simulink model "sedemo_rtos_application"  (Simulink 7.5)
settings: Solver=VariableStepDiscrete  StartTime=0.0  StopTime=19  MaxStep=inf  RelTol=1e-3
undefined symbols (not defined in the file or in its folder): des_figposition
libraries: simeventssink1 x12, simeventsgenerators1 x9, simeventsrouting1 x6, simulink x6, simeventsattributes2 x5, simeventstranslate1 x4, simeventsinfo x1, simeventsserver1 x1, simeventsqueue1 x1
settings Model: Creator=The MathWorks Inc.  ExtModeAutoUpdateStatusClock=off
settings SolverCC: InsertRTBMode=Auto
settings OptimizationCC: InitFltsAndDblsToZero=on
settings DebuggingCC: ReadBeforeWriteMsg=DisableAll  WriteAfterWriteMsg=DisableAll  WriteAfterReadMsg=DisableAll  SaveWithParameterizedLinksMsg=none  SignalResolutionControl=TryResolveAllWithWarning  MultiTaskDSMMsg=warning  MultiTaskCondExecSysMsg=none  StrictBusMsg=Warning
settings RTWCC: IncludeERTFirstTime=on
settings GRTTargetCC: TargetFcnLib=ansi_tfl_tmw.mat
settings SimEventsCC: propDiagAttribOutput=1  propDiagFcnCallOutput=1  propDiagStatOutput=0

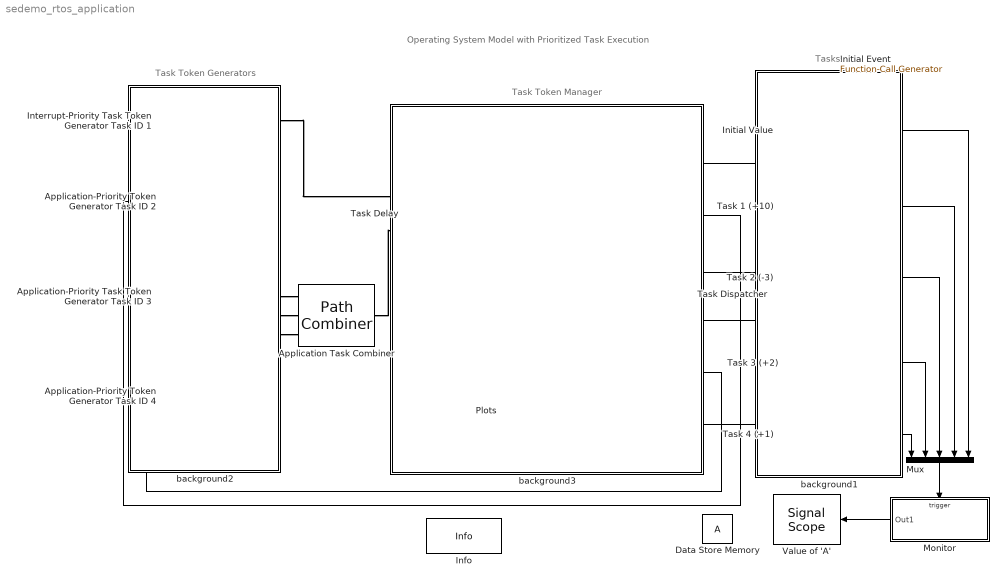
== system sedemo_rtos_application ==
  note: Operating System Model with Prioritized Task Execution
  note: Task Token Generators
  note: Task Token Manager
  note: Tasks
  Application Task Combiner : simeventsrouting1/Path Combiner  Priority=1  SystemSampleTime=-1  NumberInputPorts=3  InputPortPrecedence=IN1 port  InitialSeed=45675  SpecifyEventPriority=off  PriorityPathCombinerPortPrecedenceSelection=4100  StatNumberDeparted=Off  StatLastArrivalPort=Off  EvaluatedNumPorts=3
  Application-Priority Token Generator Task ID 2 : Subsystem
  Application-Priority Token Generator Task ID 4 : Subsystem
  Application-Priority Task Token Generator Task ID 3 : Subsystem
  Data Store Memory : DataStoreMemory  DataStoreName=A  ReadBeforeWriteMsg=warning  WriteAfterWriteMsg=warning  WriteAfterReadMsg=warning  OutDataType=sfix(16)  OutScaling=2^0
  Info : simeventsinfo/Info  SystemSampleTime=-1
  Initial Event : simulink/Ports & Subsystems/Function-Call Generator  sample_time=1e20  numberOfIterations=1
  Initial Value : Subsystem  TreatAsAtomicUnit=on
  Interrupt-Priority Task Token Generator Task ID 1 : Subsystem
  Monitor : Subsystem  TreatAsAtomicUnit=on
      settings: PropExecContextOutsideSubsystem=on
  Mux : Mux  Inputs=5
  Plots : Subsystem
  Task 1 (+10) : Subsystem  TreatAsAtomicUnit=on
  Task 2 (-3) : Subsystem  TreatAsAtomicUnit=on
  Task 3 (+2) : Subsystem  TreatAsAtomicUnit=on
  Task 4 (+1) : Subsystem  TreatAsAtomicUnit=on
  Task Delay : Subsystem
  Task Dispatcher : Subsystem
  Value of 'A' : simeventssink1/Signal Scope  Priority=1  SystemSampleTime=-1  PlotType=Stair  InputType=Signal  NumInputs=1  AttributeNameY=Count  XInputOptionSignal=Event time  XInputOptionEntity=Event time  AttributeNameX=Count  EnableEntityOutport=on  XMin=0  XMax=15.5  XLimitExceededOption=Stretch axis limits  YLimitExceededOption=Stretch axis limits  AxisGrid=on  AxisLegend=off  LineDisables=""  LineColors=b  LineStyles=-  LineMarkers=.  OpenScopeAtSimStart=on  Title=Value of 'A'  YLabel='A'  XLabel=Time  FigurePosition=des_figposition([74 15 24 20])  AxisZoom=off  DataStoreOption=Limited  DataPointsLimit=10000  StatNumberArrived=Off  ShowCountPlotted=off  ShowToolbar=off
      settings: YMin=-0.25  YMax=27
  background1 : Subsystem
      mask Display: disp('')
  background2 : Subsystem
      mask Display: disp('')
  background3 : Subsystem
      mask Display: disp('')
  wires:
  Task Dispatcher/3(Task 2) -> Task 2 (-3)/Trigger
  Task Dispatcher/4(Task 3) -> Task 3 (+2)/Trigger
  Mux/1 -> Monitor/Trigger
  Task 3 (+2)/1(Out1) -> Mux/2
  Task 2 (-3)/1(Out1) -> Mux/3
  Task 1 (+10)/1(Out1) -> Mux/4
  Task 4 (+1)/1(Out1) -> Mux/1
  Initial Value/1(Out1) -> Mux/5
  Task Dispatcher/2(Next task 1) -> Application-Priority Token Generator Task ID 2/1(Start)
  Initial Event/1 -> Initial Value/Trigger
  Task Dispatcher/1(Task 1) -> Task 1 (+10)/Trigger
  Task Dispatcher/6(Task 4) -> Task 4 (+1)/Trigger
  Task Dispatcher/5(Next task 3) -> Application-Priority Token Generator Task ID 4/1(Start)
  Monitor/1(Out1) -> Value of 'A'/1
  connections:
  Interrupt-Priority Task Token Generator Task ID 1/RConn1 -- Task Delay/LConn1
  Application-Priority Token Generator Task ID 2/RConn1 -- Application Task Combiner/LConn3
  Task Dispatcher/LConn2 -- Plots/LConn1
  Task Delay/RConn1 -- Task Dispatcher/LConn1
  Application-Priority Task Token Generator Task ID 3/RConn1 -- Application Task Combiner/LConn1
  Application-Priority Token Generator Task ID 4/RConn1 -- Application Task Combiner/LConn2
  Application Task Combiner/RConn1 -- Task Delay/LConn2

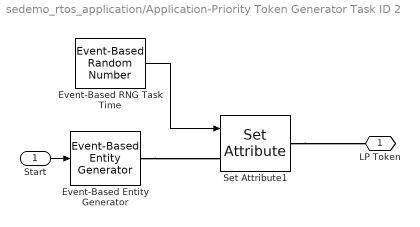
== system sedemo_rtos_application/Application-Priority Token Generator Task ID 2 ==
  Start : Inport  OutDataType=sfix(16)  OutScaling=2^0
  Event-Based Entity Generator : simeventsgenerators1/Entity Generators/Event-Based Entity Generator  Priority=1  DialogController=des_ddg_create  DialogControllerArgs=DataTag2  SystemSampleTime=-1  GenerateEntitiesUpon=Function call from port fcn  SignalEdgeType=Rising  SpecifyEventPriority=on  PriorityEntityGeneration=301  GenerateEntityAtSimulationStart=on  AllowBlocking=on  ResponseDuringBlockage=Discard generated entities  EntityType=Standard  StatNumberDeparted=Off  StatPendingEntity=Off  StatAverageIntergenerationTime=Off
  Event-Based RNG Task Time : simeventsgenerators1/Signal Generators/Event-Based Random Number  SystemSampleTime=-1  distribution=Uniform  meanExp=2  minUnif=1  maxUnif=1  pOneBern=0.25  pSuccessBino=0.5  numTrialBino=1  meanNorm=0  stdNorm=1  minTri=1  maxTri=3  modeTri=2  thresholdLogn=0  scaleLogn=1  shapeLogn=1  pSuccessGeo=0.5  meanPoiss=1  thresholdLogl=0  scaleLogl=1  thresholdGam=0  scaleGam=1  shapeGam=1  minBeta=0  maxBeta=1  shape1Beta=1  shape2Beta=1  minUnid=0  maxUnid=1  numValueUnid=2  thresholdWbl=0  scaleWbl=1  shapeWbl=1  valueVecCont=[0 1]  cdfVecCont=[0 1]  valueVecDisc=[0 1]  probVecDisc=[0.5 0.5]  seed=2354676  IsProcessed=on  isConnected=1
  Set Attribute1 : simeventsattributes2/Set Attribute  Priority=1  DialogController=des_ddg_create  DialogControllerArgs=DataTag4  SystemSampleTime=-1  AttributeFrom=Dialog|Signal port|Dialog|Dialog  AttributeName=PriorityAttributeName|TaskExecTime|TaskType|TaskID  AttributeTreatAsVector=1|1|1|1  AttributeValue=2|1|2|2  AttributeCreate=on  StatNumberDeparted=Off  EvaluatedAttributeValue={2;[];2;2}
  LP Token : PMIOPort  Port=1  Side=Right
  wires:
  Event-Based RNG Task Time/1 -> Set Attribute1/1
  Start/1 -> Event-Based Entity Generator/1
  connections:
  Event-Based Entity Generator/RConn1 -- Set Attribute1/LConn1
  Set Attribute1/RConn1 -- LP Token/RConn1

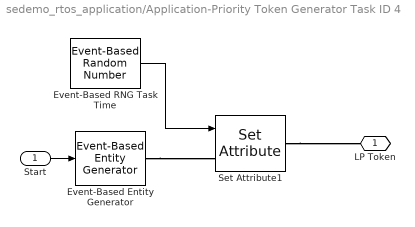
== system sedemo_rtos_application/Application-Priority Token Generator Task ID 4 ==
  Start : Inport  OutDataType=sfix(16)  OutScaling=2^0
  Event-Based Entity Generator : simeventsgenerators1/Entity Generators/Event-Based Entity Generator  Priority=1  DialogController=des_ddg_create  DialogControllerArgs=DataTag6  SystemSampleTime=-1  GenerateEntitiesUpon=Function call from port fcn  SignalEdgeType=Rising  SpecifyEventPriority=on  PriorityEntityGeneration=299  GenerateEntityAtSimulationStart=on  AllowBlocking=on  ResponseDuringBlockage=Discard generated entities  EntityType=Standard  StatNumberDeparted=Off  StatPendingEntity=Off  StatAverageIntergenerationTime=Off
  Event-Based RNG Task Time : simeventsgenerators1/Signal Generators/Event-Based Random Number  SystemSampleTime=-1  distribution=Uniform  meanExp=2  minUnif=2  maxUnif=2  pOneBern=0.25  pSuccessBino=0.5  numTrialBino=1  meanNorm=0  stdNorm=1  minTri=1  maxTri=3  modeTri=2  thresholdLogn=0  scaleLogn=1  shapeLogn=1  pSuccessGeo=0.5  meanPoiss=1  thresholdLogl=0  scaleLogl=1  thresholdGam=0  scaleGam=1  shapeGam=1  minBeta=0  maxBeta=1  shape1Beta=1  shape2Beta=1  minUnid=0  maxUnid=1  numValueUnid=2  thresholdWbl=0  scaleWbl=1  shapeWbl=1  valueVecCont=[0 1]  cdfVecCont=[0 1]  valueVecDisc=[0 1]  probVecDisc=[0.5 0.5]  seed=675409  IsProcessed=on  isConnected=1
  Set Attribute1 : simeventsattributes2/Set Attribute  Priority=1  DialogController=des_ddg_create  DialogControllerArgs=DataTag8  SystemSampleTime=-1  AttributeFrom=Dialog|Signal port|Dialog|Dialog  AttributeName=PriorityAttributeName|TaskExecTime|TaskType|TaskID  AttributeTreatAsVector=1|1|1|1  AttributeValue=4|1|2|4  AttributeCreate=on  StatNumberDeparted=Off  EvaluatedAttributeValue={4;[];2;4}
  LP Token : PMIOPort  Port=1  Side=Right
  wires:
  Event-Based RNG Task Time/1 -> Set Attribute1/1
  Start/1 -> Event-Based Entity Generator/1
  connections:
  Event-Based Entity Generator/RConn1 -- Set Attribute1/LConn1
  Set Attribute1/RConn1 -- LP Token/RConn1

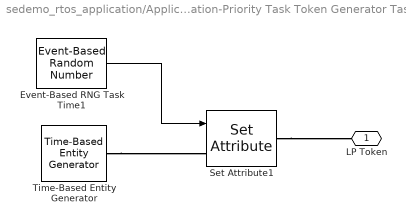
== system sedemo_rtos_application/Application-Priority Task Token Generator Task ID 3 ==
  Event-Based RNG Task Time1 : simeventsgenerators1/Signal Generators/Event-Based Random Number  SystemSampleTime=-1  distribution=Uniform  meanExp=2  minUnif=1.5  maxUnif=1.5  pOneBern=0.25  pSuccessBino=0.5  numTrialBino=1  meanNorm=0  stdNorm=1  minTri=1  maxTri=3  modeTri=2  thresholdLogn=0  scaleLogn=1  shapeLogn=1  pSuccessGeo=0.5  meanPoiss=1  thresholdLogl=0  scaleLogl=1  thresholdGam=0  scaleGam=1  shapeGam=1  minBeta=0  maxBeta=1  shape1Beta=1  shape2Beta=1  minUnid=0  maxUnid=1  numValueUnid=2  thresholdWbl=0  scaleWbl=1  shapeWbl=1  valueVecCont=[0 1]  cdfVecCont=[0 1]  valueVecDisc=[0 1]  probVecDisc=[0.5 0.5]  seed=6532180  IsProcessed=on  isConnected=1
  Set Attribute1 : simeventsattributes2/Set Attribute  Priority=1  DialogController=des_ddg_create  DialogControllerArgs=DataTag10  SystemSampleTime=-1  AttributeFrom=Dialog|Signal port|Dialog|Dialog  AttributeName=PriorityAttributeName|TaskExecTime|TaskType|TaskID  AttributeTreatAsVector=1|1|1|1  AttributeValue=3|1|2|3  AttributeCreate=on  StatNumberDeparted=Off  EvaluatedAttributeValue={3;[];2;3}
  Time-Based Entity Generator : simeventsgenerators1/Entity Generators/Time-Based Entity Generator  Priority=1  DialogController=des_ddg_create  DialogControllerArgs=DataTag12  SystemSampleTime=-1  GenerateEntitiesUpon=Intergeneration time from dialog  Distribution=Constant  Minimum=9.9  Maximum=10.5  Mean=10  InitialSeed=12345  Period=9.9  PriorityEntityGeneration=290  GenerateEntityAtSimulationStart=on  ResponseWhenBlocked=Pause generation  ResponseWhenUnblocked=Immediate restart  EntityType=Standard  StatNumberDeparted=Off  StatPendingEntity=Off  StatAverageIntergenerationTime=Off
  LP Token : PMIOPort  Port=1  Side=Right
  wires:
  Event-Based RNG Task Time1/1 -> Set Attribute1/1
  connections:
  Time-Based Entity Generator/RConn1 -- Set Attribute1/LConn1
  Set Attribute1/RConn1 -- LP Token/RConn1

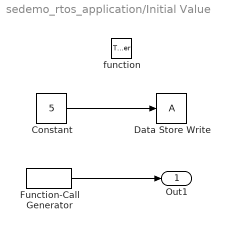
== system sedemo_rtos_application/Initial Value ==
  function : TriggerPort  TriggerType=function-call
  Constant : Constant  Value=5  OutDataType=sfix(16)  OutScaling=2^0
  Data Store Write : DataStoreWrite  DataStoreName=A  SampleTime=-1
  Function-Call Generator : simulink/Ports & Subsystems/Function-Call Generator  sample_time=-1  numberOfIterations=1
  Out1 : Outport  OutDataType=sfix(16)  OutScaling=2^0
  wires:
  Constant/1 -> Data Store Write/1
  Function-Call Generator/1 -> Out1/1

== system sedemo_rtos_application/Interrupt-Priority Task Token Generator Task ID 1 ==
  Event-Based RNG Task Time : simeventsgenerators1/Signal Generators/Event-Based Random Number  SystemSampleTime=-1  distribution=Uniform  meanExp=0.9  minUnif=.45  maxUnif=.45  pOneBern=0.25  pSuccessBino=0.5  numTrialBino=1  meanNorm=0  stdNorm=1  minTri=1  maxTri=3  modeTri=2  thresholdLogn=0  scaleLogn=1  shapeLogn=1  pSuccessGeo=0.5  meanPoiss=1  thresholdLogl=0  scaleLogl=1  thresholdGam=0  scaleGam=1  shapeGam=1  minBeta=0  maxBeta=1  shape1Beta=1  shape2Beta=1  minUnid=0  maxUnid=1  numValueUnid=2  thresholdWbl=0  scaleWbl=1  shapeWbl=1  valueVecCont=[0 1]  cdfVecCont=[0 1]  valueVecDisc=[0 1]  probVecDisc=[0.5 0.5]  seed=25899  IsProcessed=on  isConnected=1
  Set Attribute : simeventsattributes2/Set Attribute  Priority=1  DialogController=des_ddg_create  DialogControllerArgs=DataTag14  SystemSampleTime=-1  AttributeFrom=Dialog|Signal port|Dialog|Dialog  AttributeName=PriorityAttributeName|TaskExecTime|TaskType|TaskID  AttributeTreatAsVector=1|1|1|1  AttributeValue=1|1|2|1  AttributeCreate=on  StatNumberDeparted=Off  EvaluatedAttributeValue={1;[];2;1}
  Time-Based Entity Generator : simeventsgenerators1/Entity Generators/Time-Based Entity Generator  Priority=1  DialogController=des_ddg_create  DialogControllerArgs=DataTag16  SystemSampleTime=-1  GenerateEntitiesUpon=Intergeneration time from dialog  Distribution=Constant  Minimum=0  Maximum=1  Mean=1  InitialSeed=12345  Period=10  PriorityEntityGeneration=1  GenerateEntityAtSimulationStart=on  ResponseWhenBlocked=Pause generation  ResponseWhenUnblocked=Immediate restart  EntityType=Standard  StatNumberDeparted=Off  StatPendingEntity=Off  StatAverageIntergenerationTime=Off
  HP Token : PMIOPort  Port=1  Side=Right
  wires:
  Event-Based RNG Task Time/1 -> Set Attribute/1
  connections:
  Set Attribute/RConn1 -- HP Token/RConn1
  Time-Based Entity Generator/RConn1 -- Set Attribute/LConn1

== system sedemo_rtos_application/Monitor ==
  function : TriggerPort  TriggerType=function-call
  Data Store Read : DataStoreRead  DataStoreName=A  SampleTime=-1
  Out1 : Outport  OutDataType=sfix(16)  OutScaling=2^0
  wires:
  Data Store Read/1 -> Out1/1

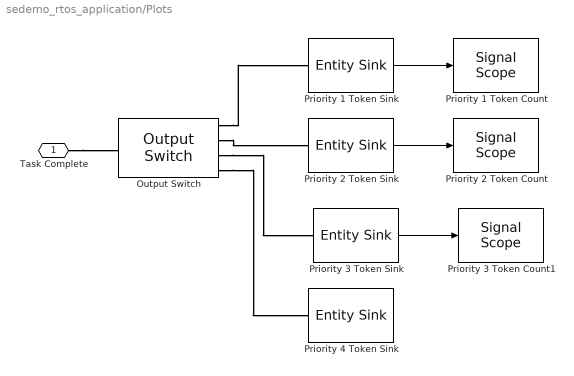
== system sedemo_rtos_application/Plots ==
  Output Switch : simeventsrouting1/Output Switch  Priority=1  SystemSampleTime=-1  NumberOutputPorts=4  SwitchingCriterion=From attribute  InitialSeed=34567  AttributeName=PriorityAttributeName  InitialConditionsOpt=off  InitialConditions=1  EntityBufferOpt=off  SpecifyEventPriority=off  PriorityOutputSwitchSelectPort=4100  TimeoutPortOpt=off  StatNumberDeparted=Off  StatNumberTimedOut=Off  StatPendingEntity=Off  StatLastDeparturePort=Off  EvaluatedNumPorts=4
  Priority 1 Token Count : simeventssink1/Signal Scope  Priority=1  SystemSampleTime=-1  PlotType=Stair  InputType=Signal  NumInputs=1  AttributeNameY=Count  XInputOptionSignal=Event time  XInputOptionEntity=Event time  AttributeNameX=Count  EnableEntityOutport=on  XMin=0  XMax=25  XLimitExceededOption=Stretch axis limits  YLimitExceededOption=Stretch axis limits  AxisGrid=on  AxisLegend=off  LineDisables=""  LineColors=b  LineStyles=-  LineMarkers=.  OpenScopeAtSimStart=off  Title=Priority 1 Tasks Completed  YLabel=Number of Tasks  XLabel=Time  FigurePosition=[759 602 303 160]  AxisZoom=off  DataStoreOption=Limited  DataPointsLimit=10000  StatNumberArrived=Off  ShowCountPlotted=off  ShowToolbar=off
      settings: YMin=0  YMax=32
  Priority 1 Token Sink : simeventssink1/Entity Sink  Priority=1  SystemSampleTime=-1  AvailableForArrivals=on  StatNumberArrived=On
  Priority 2 Token Count : simeventssink1/Signal Scope  Priority=1  SystemSampleTime=-1  PlotType=Stair  InputType=Signal  NumInputs=1  AttributeNameY=Count  XInputOptionSignal=Event time  XInputOptionEntity=Event time  AttributeNameX=Count  EnableEntityOutport=on  XMin=0  XMax=50  XLimitExceededOption=Stretch axis limits  YLimitExceededOption=Stretch axis limits  AxisGrid=on  AxisLegend=off  LineDisables=""  LineColors=b  LineStyles=-  LineMarkers=.  OpenScopeAtSimStart=off  Title=Priority 2 Tasks Completed  YLabel=Number of Tasks  XLabel=Time  FigurePosition=[759 382 300 171]  AxisZoom=off  DataStoreOption=Limited  DataPointsLimit=10000  StatNumberArrived=Off  ShowCountPlotted=off  ShowToolbar=off
      settings: YMin=0  YMax=15
  "Priority 2 Token Sink " : simeventssink1/Entity Sink  Priority=1  SystemSampleTime=-1  AvailableForArrivals=on  StatNumberArrived=On
  Priority 3 Token Count1 : simeventssink1/Signal Scope  Priority=1  SystemSampleTime=-1  PlotType=Stair  InputType=Signal  NumInputs=1  AttributeNameY=Count  XInputOptionSignal=Event time  XInputOptionEntity=Event time  AttributeNameX=Count  EnableEntityOutport=on  XMin=0  XMax=50  XLimitExceededOption=Stretch axis limits  YLimitExceededOption=Stretch axis limits  AxisGrid=on  AxisLegend=off  LineDisables=""  LineColors=b  LineStyles=-  LineMarkers=.  OpenScopeAtSimStart=off  Title=Priority 3 Tasks Completed  YLabel=Number of Tasks  XLabel=Time  FigurePosition=[756 142 299 187]  AxisZoom=off  DataStoreOption=Limited  DataPointsLimit=10000  StatNumberArrived=Off  ShowCountPlotted=off  ShowToolbar=off
      settings: YMin=0  YMax=15
  Priority 3 Token Sink : simeventssink1/Entity Sink  Priority=1  SystemSampleTime=-1  AvailableForArrivals=on  StatNumberArrived=On
  Priority 4 Token Sink : simeventssink1/Entity Sink  Priority=1  SystemSampleTime=-1  AvailableForArrivals=on  StatNumberArrived=Off
  Task Complete : PMIOPort  Port=1  Side=Left
  wires:
  Priority 1 Token Sink/1 -> Priority 1 Token Count/1
  "Priority 2 Token Sink "/1 -> Priority 2 Token Count/1
  Priority 3 Token Sink/1 -> Priority 3 Token Count1/1
  connections:
  Task Complete/RConn1 -- Output Switch/LConn1
  Output Switch/RConn1 -- Priority 1 Token Sink/LConn1
  Output Switch/RConn2 -- "Priority 2 Token Sink "/LConn1
  Output Switch/RConn3 -- Priority 3 Token Sink/LConn1
  Output Switch/RConn4 -- Priority 4 Token Sink/LConn1

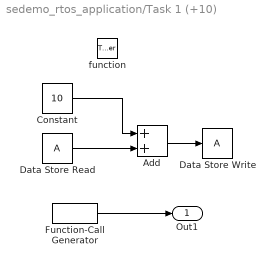
== system sedemo_rtos_application/Task 1 (+10) ==
  function : TriggerPort  TriggerType=function-call
  Add : Sum  OutDataType=sfix(16)  OutScaling=2^-10
  Constant : Constant  Value=10  OutDataType=sfix(16)  OutScaling=2^0
  Data Store Read : DataStoreRead  DataStoreName=A  SampleTime=-1
  Data Store Write : DataStoreWrite  DataStoreName=A  SampleTime=-1
  Function-Call Generator : simulink/Ports & Subsystems/Function-Call Generator  sample_time=-1  numberOfIterations=1
  Out1 : Outport  OutDataType=sfix(16)  OutScaling=2^0
  wires:
  Add/1 -> Data Store Write/1
  Constant/1 -> Add/1
  Data Store Read/1 -> Add/2
  Function-Call Generator/1 -> Out1/1

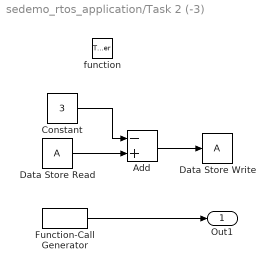
== system sedemo_rtos_application/Task 2 (-3) ==
  function : TriggerPort  TriggerType=function-call
  Add : Sum  Inputs=-+  OutDataType=sfix(16)  OutScaling=2^-10
  Constant : Constant  Value=3  OutDataType=sfix(16)  OutScaling=2^0
  Data Store Read : DataStoreRead  DataStoreName=A  SampleTime=-1
  Data Store Write : DataStoreWrite  DataStoreName=A  SampleTime=-1
  Function-Call Generator : simulink/Ports & Subsystems/Function-Call Generator  sample_time=-1  numberOfIterations=1
  Out1 : Outport  OutDataType=sfix(16)  OutScaling=2^0
  wires:
  Add/1 -> Data Store Write/1
  Constant/1 -> Add/1
  Data Store Read/1 -> Add/2
  Function-Call Generator/1 -> Out1/1

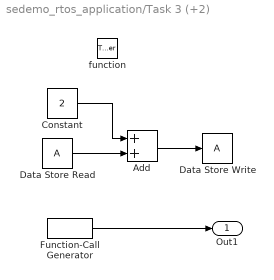
== system sedemo_rtos_application/Task 3 (+2) ==
  function : TriggerPort  TriggerType=function-call
  Add : Sum  OutDataType=sfix(16)  OutScaling=2^-10
  Constant : Constant  Value=2  OutDataType=sfix(16)  OutScaling=2^0
  Data Store Read : DataStoreRead  DataStoreName=A  SampleTime=-1
  Data Store Write : DataStoreWrite  DataStoreName=A  SampleTime=-1
  Function-Call Generator : simulink/Ports & Subsystems/Function-Call Generator  sample_time=-1  numberOfIterations=1
  Out1 : Outport  OutDataType=sfix(16)  OutScaling=2^0
  wires:
  Add/1 -> Data Store Write/1
  Constant/1 -> Add/1
  Data Store Read/1 -> Add/2
  Function-Call Generator/1 -> Out1/1

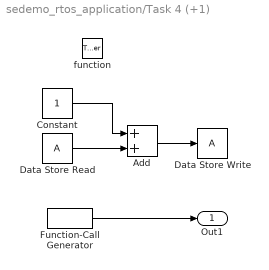
== system sedemo_rtos_application/Task 4 (+1) ==
  function : TriggerPort  TriggerType=function-call
  Add : Sum  OutDataType=sfix(16)  OutScaling=2^-10
  Constant : Constant  OutDataType=sfix(16)  OutScaling=2^0
  Data Store Read : DataStoreRead  DataStoreName=A  SampleTime=-1
  Data Store Write : DataStoreWrite  DataStoreName=A  SampleTime=-1
  Function-Call Generator : simulink/Ports & Subsystems/Function-Call Generator  sample_time=-1  numberOfIterations=1
  Out1 : Outport  OutDataType=sfix(16)  OutScaling=2^0
  wires:
  Add/1 -> Data Store Write/1
  Constant/1 -> Add/1
  Data Store Read/1 -> Add/2
  Function-Call Generator/1 -> Out1/1

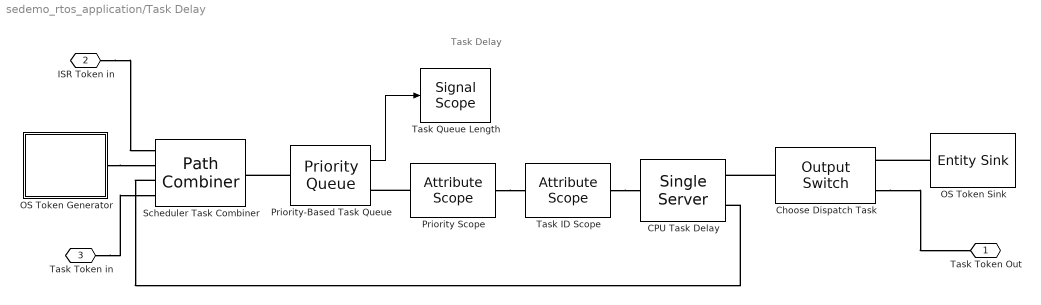
== system sedemo_rtos_application/Task Delay ==
  note: Task Delay
  CPU Task Delay : simeventsserver1/Single Server  Priority=1  SystemSampleTime=-1  ServiceTimeFrom=Attribute  ServiceTime=0.5  AttributeName=TaskExecTime  PriorityServiceCompletion=4  PermitPreemption=on  SortingAttributeName=PriorityAttributeName  SortingDirection=Ascending  WriteToAttribute=on  ResidualAttributeName=TaskExecTime  CreateAttribute=off  EnableTOPort=off  StatNumberDeparted=Off  StatNumberInBlock=Off  StatNumberPreempted=Off  StatPendingEntity=Off  StatAverageWait=Off  StatUtilization=Off  StatNumberTimedout=Off
  Choose Dispatch Task : simeventsrouting1/Output Switch  Priority=1  SystemSampleTime=-1  NumberOutputPorts=2  SwitchingCriterion=From attribute  InitialSeed=34567  AttributeName=TaskType  InitialConditionsOpt=off  InitialConditions=1  EntityBufferOpt=off  SpecifyEventPriority=off  PriorityOutputSwitchSelectPort=4100  TimeoutPortOpt=off  StatNumberDeparted=Off  StatNumberTimedOut=Off  StatPendingEntity=Off  StatLastDeparturePort=Off  EvaluatedNumPorts=2
  OS Token Generator : Subsystem
  OS Token Sink : simeventssink1/Entity Sink  Priority=1  SystemSampleTime=-1  AvailableForArrivals=on  StatNumberArrived=Off
  Priority Scope : simeventssink1/Attribute Scope  Priority=1  SystemSampleTime=-1  PlotType=Stair  InputType=Attribute  NumInputs=1  AttributeNameY=PriorityAttributeName  XInputOptionSignal=Event time  XInputOptionEntity=Event time  AttributeNameX=Count  EnableEntityOutport=on  XMin=0  XMax=15.5  XLimitExceededOption=Stretch axis limits  YLimitExceededOption=Stretch axis limits  AxisGrid=on  AxisLegend=off  LineDisables=""  LineColors=b  LineStyles=-  LineMarkers=.  OpenScopeAtSimStart=on  Title=Priority Value for Tasks  YLabel=Priority  XLabel=Time  FigurePosition=des_figposition([2 15 24 20])  AxisZoom=off  DataStoreOption=Limited  DataPointsLimit=10000  StatNumberArrived=Off  ShowCountPlotted=off  ShowToolbar=off
      settings: YMin=0  YMax=6
  Priority-Based Task Queue : simeventsqueue1/Priority Queue  Priority=1  SystemSampleTime=-1  Capacity=inf  SortingAttributeName=PriorityAttributeName  SortingDirection=Ascending  EnableTOPort=off  StatNumberDeparted=Off  StatNumberInBlock=On  StatPendingEntity=Off  StatAverageWait=Off  StatAverageQueueLength=Off  StatNumberTimedout=Off
  Scheduler Task Combiner : simeventsrouting1/Path Combiner  Priority=1  SystemSampleTime=-1  NumberInputPorts=4  InputPortPrecedence=IN1 port  InitialSeed=45675  SpecifyEventPriority=off  PriorityPathCombinerPortPrecedenceSelection=4100  StatNumberDeparted=Off  StatLastArrivalPort=Off  EvaluatedNumPorts=4
  Task ID Scope : simeventssink1/Attribute Scope  Priority=1  SystemSampleTime=-1  PlotType=Stair  InputType=Attribute  NumInputs=1  AttributeNameY=TaskID  XInputOptionSignal=Event time  XInputOptionEntity=Event time  AttributeNameX=Count  EnableEntityOutport=on  XMin=0  XMax=15.5  XLimitExceededOption=Stretch axis limits  YLimitExceededOption=Stretch axis limits  AxisGrid=on  AxisLegend=off  LineDisables=""  LineColors=b  LineStyles=-  LineMarkers=.  OpenScopeAtSimStart=on  Title=Present Task ID  YLabel=Task ID  XLabel=Time  FigurePosition=des_figposition([26 15 24 20])  AxisZoom=off  DataStoreOption=Limited  DataPointsLimit=10000  StatNumberArrived=Off  ShowCountPlotted=off  ShowToolbar=off
      settings: YMin=0  YMax=4
  Task Queue Length : simeventssink1/Signal Scope  Priority=1  SystemSampleTime=-1  PlotType=Stair  InputType=Signal  NumInputs=1  AttributeNameY=Count  XInputOptionSignal=Event time  XInputOptionEntity=Event time  AttributeNameX=Count  EnableEntityOutport=on  XMin=0  XMax=15.5  XLimitExceededOption=Stretch axis limits  YLimitExceededOption=Stretch axis limits  AxisGrid=on  AxisLegend=off  LineDisables=""  LineColors=b  LineStyles=-  LineMarkers=.  OpenScopeAtSimStart=on  Title=Task Queue Length  YLabel=Queue Length  XLabel=Time  FigurePosition=des_figposition([50 15 24 20])  AxisZoom=off  DataStoreOption=Limited  DataPointsLimit=10000  StatNumberArrived=Off  ShowCountPlotted=off  ShowToolbar=off
      settings: YMin=0  YMax=3
  Task Token Out : PMIOPort  Port=1  Side=Right
  ISR Token in : PMIOPort  Port=2  Side=Left
  Task Token in : PMIOPort  Port=3  Side=Left
  wires:
  Priority-Based Task Queue/1 -> Task Queue Length/1
  connections:
  Priority-Based Task Queue/LConn1 -- Scheduler Task Combiner/RConn1
  Priority Scope/LConn1 -- Priority-Based Task Queue/RConn1
  Choose Dispatch Task/LConn1 -- CPU Task Delay/RConn1
  OS Token Sink/LConn1 -- Choose Dispatch Task/RConn1
  ISR Token in/RConn1 -- Scheduler Task Combiner/LConn1
  Priority Scope/RConn1 -- Task ID Scope/LConn1
  Task ID Scope/RConn1 -- CPU Task Delay/LConn1
  Scheduler Task Combiner/LConn3 -- CPU Task Delay/RConn2
  Choose Dispatch Task/RConn2 -- Task Token Out/RConn1
  OS Token Generator/RConn1 -- Scheduler Task Combiner/LConn2
  Task Token in/RConn1 -- Scheduler Task Combiner/LConn4

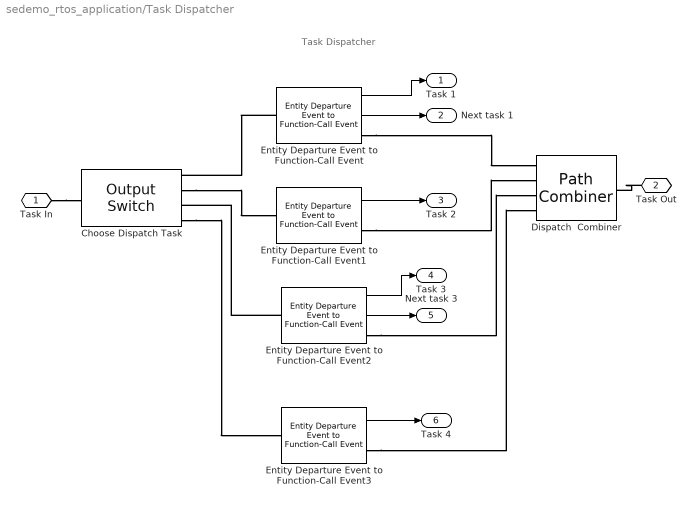
== system sedemo_rtos_application/Task Dispatcher ==
  note: Task Dispatcher
  Choose Dispatch Task : simeventsrouting1/Output Switch  Priority=1  SystemSampleTime=-1  NumberOutputPorts=4  SwitchingCriterion=From attribute  InitialSeed=34567  AttributeName=TaskID  InitialConditionsOpt=off  InitialConditions=1  EntityBufferOpt=off  SpecifyEventPriority=off  PriorityOutputSwitchSelectPort=4100  TimeoutPortOpt=off  StatNumberDeparted=Off  StatNumberTimedOut=Off  StatPendingEntity=Off  StatLastDeparturePort=Off  EvaluatedNumPorts=4
  Dispatch  Combiner : simeventsrouting1/Path Combiner  Priority=1  SystemSampleTime=-1  NumberInputPorts=4  InputPortPrecedence=IN1 port  InitialSeed=45675  SpecifyEventPriority=off  PriorityPathCombinerPortPrecedenceSelection=4100  StatNumberDeparted=Off  StatLastArrivalPort=Off  EvaluatedNumPorts=4
  Entity Departure Event to Function-Call Event : simeventstranslate1/Entity Departure Event to Function-Call Event  Priority=1  SystemSampleTime=-1  TimingFunctionCallF1=After entity departure  EnableE1Port=off  EnableF2Port=on  TimingFunctionCallF2=After entity departure  EnableE2Port=off  StatNumberDeparted=Off  StatNumberF1Calls=Off  StatNumberF2Calls=Off  IsInsideAFB=off
  Entity Departure Event to Function-Call Event1 : simeventstranslate1/Entity Departure Event to Function-Call Event  Priority=1  SystemSampleTime=-1  TimingFunctionCallF1=After entity departure  EnableE1Port=off  EnableF2Port=off  TimingFunctionCallF2=After entity departure  EnableE2Port=off  StatNumberDeparted=Off  StatNumberF1Calls=Off  StatNumberF2Calls=Off  IsInsideAFB=off
  Entity Departure Event to Function-Call Event2 : simeventstranslate1/Entity Departure Event to Function-Call Event  Priority=1  SystemSampleTime=-1  TimingFunctionCallF1=After entity departure  EnableE1Port=off  EnableF2Port=on  TimingFunctionCallF2=After entity departure  EnableE2Port=off  StatNumberDeparted=Off  StatNumberF1Calls=Off  StatNumberF2Calls=Off  IsInsideAFB=off
  Entity Departure Event to Function-Call Event3 : simeventstranslate1/Entity Departure Event to Function-Call Event  Priority=1  SystemSampleTime=-1  TimingFunctionCallF1=After entity departure  EnableE1Port=off  EnableF2Port=off  TimingFunctionCallF2=After entity departure  EnableE2Port=off  StatNumberDeparted=Off  StatNumberF1Calls=Off  StatNumberF2Calls=Off  IsInsideAFB=off
  Task In : PMIOPort  Port=1  Side=Left
  Task Out : PMIOPort  Port=2  Side=Left
  Task 1 : Outport  OutDataType=sfix(16)  OutScaling=2^0
  Next task 1 : Outport  Port=2  OutDataType=sfix(16)  OutScaling=2^0
  Task 2 : Outport  Port=3  OutDataType=sfix(16)  OutScaling=2^0
  Task 3 : Outport  Port=4  OutDataType=sfix(16)  OutScaling=2^0
  Next task 3 : Outport  Port=5  OutDataType=sfix(16)  OutScaling=2^0
  Task 4 : Outport  Port=6  OutDataType=sfix(16)  OutScaling=2^0
  wires:
  Entity Departure Event to Function-Call Event/2 -> Next task 1/1
  Entity Departure Event to Function-Call Event/1 -> Task 1/1
  Entity Departure Event to Function-Call Event1/1 -> Task 2/1
  Entity Departure Event to Function-Call Event2/1 -> Task 3/1
  Entity Departure Event to Function-Call Event2/2 -> Next task 3/1
  Entity Departure Event to Function-Call Event3/1 -> Task 4/1
  connections:
  Task Out/RConn1 -- Dispatch  Combiner/RConn1
  Task In/RConn1 -- Choose Dispatch Task/LConn1
  Entity Departure Event to Function-Call Event/LConn1 -- Choose Dispatch Task/RConn1
  Entity Departure Event to Function-Call Event/RConn1 -- Dispatch  Combiner/LConn1
  Choose Dispatch Task/RConn2 -- Entity Departure Event to Function-Call Event1/LConn1
  Entity Departure Event to Function-Call Event1/RConn1 -- Dispatch  Combiner/LConn2
  Entity Departure Event to Function-Call Event2/RConn1 -- Dispatch  Combiner/LConn3
  Entity Departure Event to Function-Call Event3/RConn1 -- Dispatch  Combiner/LConn4
  Entity Departure Event to Function-Call Event2/LConn1 -- Choose Dispatch Task/RConn3
  Choose Dispatch Task/RConn4 -- Entity Departure Event to Function-Call Event3/LConn1

== system sedemo_rtos_application/background1 ==

== system sedemo_rtos_application/background2 ==

== system sedemo_rtos_application/background3 ==

== system sedemo_rtos_application/Task Delay/OS Token Generator ==
  Idle Task Token Generator : simeventsgenerators1/Entity Generators/Time-Based Entity Generator  Priority=1  DialogController=des_ddg_create  DialogControllerArgs=DataTag28  SystemSampleTime=-1  GenerateEntitiesUpon=Intergeneration time from dialog  Distribution=Constant  Minimum=0  Maximum=1  Mean=1  InitialSeed=12345  Period=inf  PriorityEntityGeneration=9  GenerateEntityAtSimulationStart=on  ResponseWhenBlocked=Pause generation  ResponseWhenUnblocked=Immediate restart  EntityType=Standard  StatNumberDeparted=Off  StatPendingEntity=Off  StatAverageIntergenerationTime=Off
  Set Attribute1 : simeventsattributes2/Set Attribute  Priority=1  DialogController=des_ddg_create  DialogControllerArgs=DataTag30  SystemSampleTime=-1  AttributeFrom=Dialog|Dialog|Dialog|Dialog  AttributeName=PriorityAttributeName|TaskExecTime|TaskType|TaskID  AttributeTreatAsVector=1|1|1|1  AttributeValue=6|inf|2|0  AttributeCreate=on  StatNumberDeparted=Off  EvaluatedAttributeValue={6;inf;2;0}
  OS  Tokens : PMIOPort  Port=1  Side=Right
  connections:
  Idle Task Token Generator/RConn1 -- Set Attribute1/LConn1
  Set Attribute1/RConn1 -- OS  Tokens/RConn1
